simulink model "my_demod_test"  (R2014b)
settings: Solver=ode45  StartTime=0.0  StopTime=.4  RelTol=1e-3
libraries: siglabs_lib x2, simulink x1, commrandsrc2 x1
settings Model: Creator=Ben  LastModifiedBy=Ben

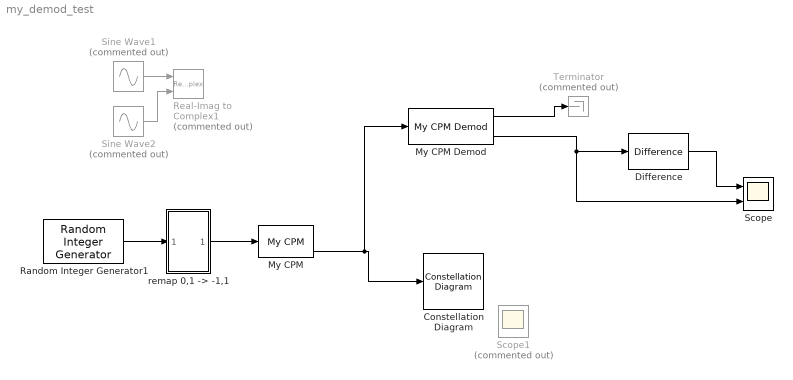
== system my_demod_test ==
  Constellation Diagram : ConstellationDiagram
  Difference : simulink/Discrete/Difference  ICPrevInput=0.0  InputProcessing=Inherited  OutMin=[]  OutMax=[]  OutDataType=fixdt(1, 16)  OutScaling=2^-10  DoSatur=off
  My CPM : siglabs_lib/My CPM  SampsPerSym=10  RotationsPerSym=1  FilterBufferLength=3  ClockUpDownFrequency=100  PatternVectorDialog=[ones(1,7)*1 ones(1,7)*2 ones(1,6)*0]  PatternVectorRepeatDialog=2
  My CPM Demod : siglabs_lib/My CPM Demod  SampsPerSym=10  RotationsPerSym=1
  Random Integer Generator1 : commrandsrc2/Random Integer Generator  mul=2  seed=42  Ts=1/(10000)  frameBased=off  sampPerFrame=1024  orient=off  outDataType=double
  Real-Imag to Complex1 : RealImagToComplex  Commented=on
  Scope : Scope  NumInputPorts=2
      settings: YMin=-8~-50  YMax=8~250
  Scope1 : Scope  Commented=on
      settings: YMin=0  YMax=12000
  Sine Wave1 : Sin  Commented=on  Frequency=20000*2*pi  Phase=2*pi*90/360  SampleTime=2.00E-06
  Sine Wave2 : Sin  Commented=on  Frequency=20000*2*pi  SampleTime=2.00E-06
  Terminator : Terminator  Commented=on
  "remap 0,1 -> -1,1" : Subsystem
  wires:
  Sine Wave1/1 -> Real-Imag to Complex1/1
  Sine Wave2/1 -> Real-Imag to Complex1/2
  My CPM Demod/1 -> Terminator/1
  My CPM Demod/2 -> Scope/2, Difference/1
  Random Integer Generator1/1 -> "remap 0,1 -> -1,1"/1(In1)
  "remap 0,1 -> -1,1"/1(Out1) -> My CPM/1
  My CPM/3 -> My CPM Demod/1, Constellation Diagram/1
  Difference/1 -> Scope/1

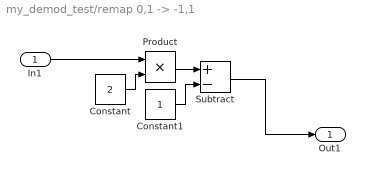
== system my_demod_test/remap 0,1 -> -1,1 ==
  In1 : Inport
  Constant : Constant  Value=2
  Constant1 : Constant
  Product : Product
  Subtract : Sum  Inputs=+-
  Out1 : Outport
  wires:
  Constant/1 -> Product/2
  In1/1 -> Product/1
  Subtract/1 -> Out1/1
  Product/1 -> Subtract/1
  Constant1/1 -> Subtract/2
